simulink model "UDPKommunikation"  (Simulink 8.6)
settings: Solver=FixedStepAuto  StartTime=0.0  StopTime=inf  FixedStep=0.1  RelTol=1e-3
libraries: xpcutilitieslib x10, xpcrtudplib x10
settings Model: Creator=atlabor  LastModifiedBy=atlabor
settings DataIOCC: SaveFormat=Dataset  SignalLoggingSaveFormat=Dataset
settings OptimizationCC: ExpressionDepthLimit=128
settings DebuggingCC: UnderspecifiedInitializationDetection=Simplified  MergeDetectMultiDrivingBlocksExec=error  SolverPrmCheckMsg=none  FcnCallInpInsideContextMsg=EnableAllAsError  StateNameClashWarn=none
settings HardwareCC: ProdBitPerPointer=64  ProdLargestAtomicFloat=Float  ProdIntDivRoundTo=Zero  ProdEndianess=LittleEndian  ProdWordSize=64  ProdHWDeviceType=Intel->x86-64 (Windows64)
settings GRTTargetCC: GeneratePreprocessorConditionals=Use local settings  CombineOutputUpdateFcns=on  GRTInterface=off

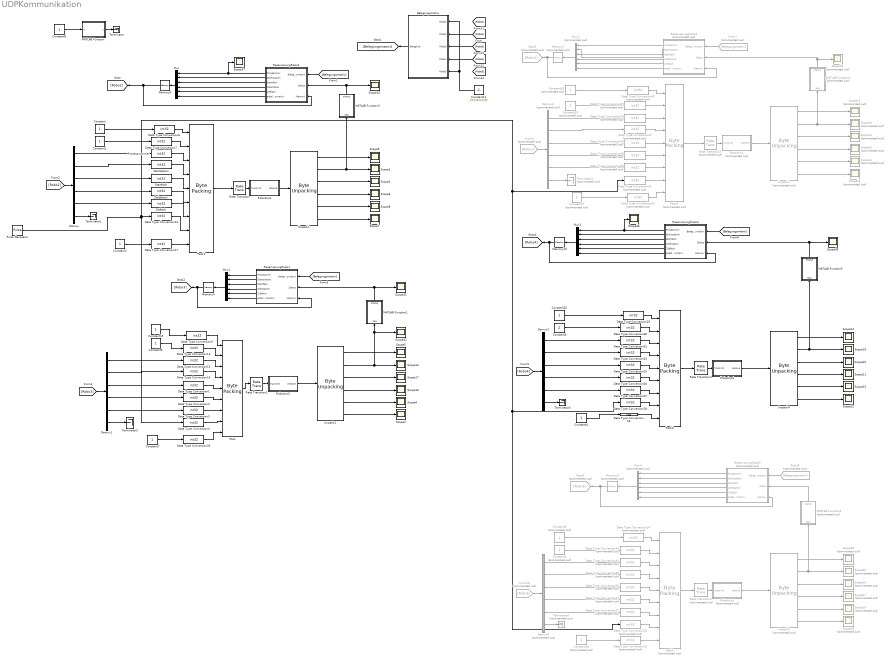
== system UDPKommunikation ==
  Belegungsmatrix : MATLAB Function  TreatAsAtomicUnit=on
  Constant{,1..2,4,7..9,15,25} (9 alike) : Constant
  Constant{5..6,10,17,28..29} (6 alike) : Constant  Commented=on
  Constant11 : Constant  Value=[0;0;0;0;0;0]
  Constant3 : Constant  Value=2
  Data Type Conversion{1..7,13..18,25..33} (22 alike) : DataTypeConversion  OutDataTypeStr=int32
  Data Type Conversion{19..24,34..45} (18 alike) : DataTypeConversion  Commented=on  OutDataTypeStr=int32
  Demux : Demux  Outputs=6
  Demux1 : Demux  Outputs=6
  Demux2 : Demux  Outputs=6
  Demux3 : Demux  Commented=on  Outputs=6
  Demux4 : Demux  Commented=on  Outputs=6
  From10 : From  Commented=on  GotoTag=Robo5
  From6 : From  Commented=on  GotoTag=Robo1
  From7 : From  Commented=on  GotoTag=Belegungsmatrix
  From9 : From  Commented=on  GotoTag=Belegungsmatrix
  Goto3 : Goto  Commented=on  GotoTag=Robo1
  Goto5 : Goto  Commented=on  GotoTag=Robo5
  MATLAB Function : MATLAB Function  TreatAsAtomicUnit=on
  MATLAB Function1 : MATLAB Function  TreatAsAtomicUnit=on
  MATLAB Function2 : MATLAB Function  Commented=on  TreatAsAtomicUnit=on
  MATLAB Function3 : MATLAB Function  TreatAsAtomicUnit=on
  MATLAB Function4 : MATLAB Function  Commented=on  TreatAsAtomicUnit=on
  MATLAB Function5 : MATLAB Function  TreatAsAtomicUnit=on
  Memory10 : Memory
  Memory4 : Memory
  Memory5 : Memory
  Memory7 : Memory  Commented=on
  Memory9 : Memory  Commented=on
  Mux : Mux  Inputs=6
  Mux1 : Mux  Inputs=6
  Mux2 : Mux  Commented=on  Inputs=6
  Mux3 : Mux  Inputs=6
  Mux4 : Mux  Commented=on  Inputs=6
  Pack : xpcutilitieslib/Byte Packing   MaskPackedDataType=uint8  MaskUnpackedDataTypes={'int32','int32','int32','int32','int32','int32','int32','int32','int32'}  MaskAlignment=1
  Pack1 : xpcutilitieslib/Byte Packing   Commented=on  MaskPackedDataType=uint8  MaskUnpackedDataTypes={'int32','int32','int32','int32','int32','int32','int32','int32','int32'}  MaskAlignment=1
  Pack2 : xpcutilitieslib/Byte Packing   MaskPackedDataType=uint8  MaskUnpackedDataTypes={'int32','int32','int32','int32','int32','int32','int32','int32','int32'}  MaskAlignment=1
  Pack3 : xpcutilitieslib/Byte Packing   MaskPackedDataType=uint8  MaskUnpackedDataTypes={'int32','int32','int32','int32','int32','int32','int32','int32','int32'}  MaskAlignment=1
  Pack4 : xpcutilitieslib/Byte Packing   Commented=on  MaskPackedDataType=uint8  MaskUnpackedDataTypes={'int32','int32','int32','int32','int32','int32','int32','int32','int32'}  MaskAlignment=1
  Prozessnummer : DataTypeConversion  OutDataTypeStr=int32
  Pulse Generator : DiscretePulseGenerator  PulseType=Time based  Amplitude=3  Period=1  PulseWidth=50
  Rate Transition : RateTransition  OutPortSampleTime=0.5
  Rate Transition1 : RateTransition  OutPortSampleTime=0.1
  Rate Transition2 : RateTransition  Commented=on  OutPortSampleTime=0.5
  Rate Transition3 : RateTransition  OutPortSampleTime=0.5
  Rate Transition4 : RateTransition  Commented=on  OutPortSampleTime=0.5
  ReservierungRobo1 : MATLAB Function  TreatAsAtomicUnit=on
  ReservierungRobo2 : MATLAB Function  TreatAsAtomicUnit=on
  ReservierungRobo3 : MATLAB Function  Commented=on  TreatAsAtomicUnit=on
  ReservierungRobo4 : MATLAB Function  TreatAsAtomicUnit=on
  ReservierungRobo5 : MATLAB Function  Commented=on  TreatAsAtomicUnit=on
  Robotino1 : Subsystem  Commented=on  TreatAsAtomicUnit=on
  Robotino2 : Subsystem  TreatAsAtomicUnit=on
  Robotino3 : Subsystem  TreatAsAtomicUnit=on
  Robotino4 : Subsystem  TreatAsAtomicUnit=on
  Robotino5 : Subsystem  Commented=on  TreatAsAtomicUnit=on
  Scope{1..9,16..24,31..33,35..37} (24 alike) : Scope
  Scope{10..15,25..30,34} (13 alike) : Scope  Commented=on
  Startfach : DataTypeConversion  OutDataTypeStr=int32
  Startstation : DataTypeConversion  OutDataTypeStr=int32
  Terminator{,1..3} (4 alike) : Terminator
  Terminator4 : Terminator  Commented=on
  Terminator5 : Terminator  Commented=on
  Unpack1 : xpcutilitieslib/Byte Unpacking   MaskUnpackedDataTypes={'uint32','uint32','uint32','uint32','uint32','uint32'}  MaskUnpackedDataSizes={1, 1,1,1,1,1}  MaskAlignment=1
  Unpack2 : xpcutilitieslib/Byte Unpacking   MaskUnpackedDataTypes={'uint32','uint32','uint32','uint32','uint32','uint32'}  MaskUnpackedDataSizes={1, 1,1,1,1,1}  MaskAlignment=1
  Unpack3 : xpcutilitieslib/Byte Unpacking   Commented=on  MaskUnpackedDataTypes={'uint32','uint32','uint32','uint32','uint32','uint32'}  MaskUnpackedDataSizes={1, 1,1,1,1,1}  MaskAlignment=1
  Unpack4 : xpcutilitieslib/Byte Unpacking   MaskUnpackedDataTypes={'uint32','uint32','uint32','uint32','uint32','uint32'}  MaskUnpackedDataSizes={1, 1,1,1,1,1}  MaskAlignment=1
  Unpack5 : xpcutilitieslib/Byte Unpacking   Commented=on  MaskUnpackedDataTypes={'uint32','uint32','uint32','uint32','uint32','uint32'}  MaskUnpackedDataSizes={1, 1,1,1,1,1}  MaskAlignment=1
  Zielfach : DataTypeConversion  OutDataTypeStr=int32
  Zielstation : DataTypeConversion  OutDataTypeStr=int32
  wires:
  Constant/1 -> Data Type Conversion6/1
  Pack2/1 -> Rate Transition/1
  Data Type Conversion6/1 -> Pack2/1
  Robotino2/1(receive) -> Unpack1/1
  Data Type Conversion7/1 -> Pack2/2
  Prozessnummer/1 -> Pack2/3
  Startstation/1 -> Pack2/4
  Startfach/1 -> Pack2/5
  Zielstation/1 -> Pack2/6
  Data Type Conversion13/1 -> Pack2/8
  Zielfach/1 -> Pack2/7
  Constant1/1 -> Data Type Conversion7/1
  Rate Transition/1 -> Robotino2/1(transmit)
  Constant8/1 -> MATLAB Function/1(u)
  MATLAB Function/1(y) -> Terminator/1
  Robotino3/1(receive) -> Unpack2/1
  Rate Transition1/1 -> Robotino3/1(transmit)
  Rate Transition2/1 -> Robotino1/1(transmit)
  Pack/1 -> Rate Transition1/1
  Data Type Conversion5/1 -> Pack/1
  Data Type Conversion14/1 -> Pack/2
  Data Type Conversion15/1 -> Pack/3
  Data Type Conversion16/1 -> Pack/4
  Data Type Conversion1/1 -> Pack/5
  Data Type Conversion2/1 -> Pack/6
  Data Type Conversion4/1 -> Pack/8
  Data Type Conversion3/1 -> Pack/7
  Constant9/1 -> Data Type Conversion14/1
  Pack4/1 -> Rate Transition2/1
  Constant15/1 -> Data Type Conversion5/1
  Rate Transition3/1 -> Robotino4/1(transmit)
  Pack3/1 -> Rate Transition3/1
  Data Type Conversion29/1 -> Pack3/1
  Data Type Conversion30/1 -> Pack3/2
  Data Type Conversion31/1 -> Pack3/3
  Data Type Conversion32/1 -> Pack3/4
  Data Type Conversion25/1 -> Pack3/5
  Data Type Conversion26/1 -> Pack3/6
  Data Type Conversion28/1 -> Pack3/8
  Data Type Conversion27/1 -> Pack3/7
  Constant25/1 -> Data Type Conversion29/1
  Constant3/1 -> Data Type Conversion30/1
  Unpack2/1 -> Scope5/1
  Unpack2/3 -> Scope17/1
  Unpack2/4 -> Scope18/1
  Unpack2/5 -> Scope4/1
  Unpack2/6 -> Scope2/1
  Data Type Conversion33/1 -> Pack/9
  Constant7/1 -> Data Type Conversion33/1
  Data Type Conversion42/1 -> Pack4/1
  Data Type Conversion35/1 -> Pack4/2
  Data Type Conversion36/1 -> Pack4/3
  Data Type Conversion37/1 -> Pack4/4
  Data Type Conversion34/1 -> Pack4/5
  Data Type Conversion38/1 -> Pack4/6
  Data Type Conversion41/1 -> Pack4/8
  Data Type Conversion39/1 -> Pack4/7
  Constant29/1 -> Data Type Conversion35/1
  Data Type Conversion40/1 -> Pack4/9
  Constant17/1 -> Data Type Conversion40/1
  Unpack1/1 -> Scope9/1
  Unpack1/2 -> MATLAB Function3/1(new), Scope1/1
  Unpack1/3 -> Scope3/1
  Unpack1/4 -> Scope6/1
  Unpack1/5 -> Scope8/1
  Unpack1/6 -> Scope7/1
  Robotino1/1(receive) -> Unpack3/1
  Unpack3/1 -> Scope15/1
  Unpack3/2 -> MATLAB Function2/1(new), Scope10/1
  Unpack3/3 -> Scope11/1
  Unpack3/4 -> Scope12/1
  Unpack3/5 -> Scope14/1
  Unpack3/6 -> Scope13/1
  Robotino4/1(receive) -> Unpack4/1
  Unpack4/1 -> Scope24/1
  Unpack4/3 -> Scope20/1
  Unpack4/4 -> Scope21/1
  Unpack4/5 -> Scope23/1
  Unpack4/6 -> Scope22/1
  Constant28/1 -> Data Type Conversion42/1
  Unpack4/2 -> MATLAB Function5/1(new), Scope19/1
  Data Type Conversion17/1 -> Pack2/9
  Constant2/1 -> Data Type Conversion17/1
  Data Type Conversion18/1 -> Pack3/9
  Constant4/1 -> Data Type Conversion18/1
  MATLAB Function3/1(status) -> ReservierungRobo2/2(Status), Scope33/1
  Rate Transition4/1 -> Robotino5/1(transmit)
  Pack1/1 -> Rate Transition4/1
  Data Type Conversion24/1 -> Pack1/1
  Data Type Conversion43/1 -> Pack1/2
  Data Type Conversion44/1 -> Pack1/3
  Data Type Conversion45/1 -> Pack1/4
  Data Type Conversion20/1 -> Pack1/5
  Data Type Conversion21/1 -> Pack1/6
  Data Type Conversion23/1 -> Pack1/8
  Data Type Conversion22/1 -> Pack1/7
  Constant5/1 -> Data Type Conversion24/1
  Constant6/1 -> Data Type Conversion43/1
  Pulse Generator/1 -> Data Type Conversion13/1, Data Type Conversion28/1, Data Type Conversion23/1, Data Type Conversion41/1, Data Type Conversion4/1
  Robotino5/1(receive) -> Unpack5/1
  Unpack5/1 -> Scope30/1
  Unpack5/3 -> Scope26/1
  Unpack5/4 -> Scope27/1
  Unpack5/5 -> Scope29/1
  Unpack5/6 -> Scope28/1
  Data Type Conversion19/1 -> Pack1/9
  Constant10/1 -> Data Type Conversion19/1
  ReservierungRobo2/1(Prozessnmr) -> Scope37/1, Mux/1
  ReservierungRobo2/2(Startstation) -> Mux/2
  ReservierungRobo2/3(Startfach) -> Mux/3
  ReservierungRobo2/4(Zielstation) -> Mux/4
  ReservierungRobo2/5(Zielfach) -> Mux/5
  ReservierungRobo2/6(enableBelegungsmatrix) -> Mux/6
  Belegungsmatrix/1(BelegOut) -> [Belegungsmatrix]
  [Belegungsmatrix] -> ReservierungRobo2/1(Belegungsmatrix)
  [Robo2] -> Demux/1
  Demux/1 -> Prozessnummer/1
  Demux/2 -> Startstation/1
  Demux/3 -> Startfach/1
  Demux/4 -> Zielstation/1
  Demux/5 -> Zielfach/1
  Demux/6 -> Terminator1/1
  Unpack2/2 -> MATLAB Function1/1(new), Scope32/1, Scope16/1
  ReservierungRobo1/1(Prozessnmr) -> Mux1/1
  ReservierungRobo1/2(Startstation) -> Mux1/2
  ReservierungRobo1/3(Startfach) -> Mux1/3
  ReservierungRobo1/4(Zielstation) -> Mux1/4
  ReservierungRobo1/5(Zielfach) -> Mux1/5
  ReservierungRobo1/6(enableBelegungsmatrix) -> Mux1/6
  [Belegungsmatrix] -> ReservierungRobo1/1(Belegungsmatrix)
  [Robo3] -> Demux1/1
  Demux1/1 -> Data Type Conversion15/1
  Demux1/2 -> Data Type Conversion16/1
  Demux1/3 -> Data Type Conversion1/1
  Demux1/4 -> Data Type Conversion2/1
  Demux1/5 -> Data Type Conversion3/1
  Demux1/6 -> Terminator2/1
  [Robo4] -> Demux2/1
  Demux2/1 -> Data Type Conversion31/1
  Demux2/2 -> Data Type Conversion32/1
  Demux2/3 -> Data Type Conversion25/1
  Demux2/4 -> Data Type Conversion26/1
  Demux2/5 -> Data Type Conversion27/1
  Demux2/6 -> Terminator3/1
  From6/1 -> Demux3/1
  Demux3/1 -> Data Type Conversion36/1
  Demux3/2 -> Data Type Conversion37/1
  Demux3/3 -> Data Type Conversion34/1
  Demux3/4 -> Data Type Conversion38/1
  Demux3/5 -> Data Type Conversion39/1
  Demux3/6 -> Terminator4/1
  MATLAB Function2/1(status) -> ReservierungRobo3/2(Status), Scope34/1
  ReservierungRobo3/1(Prozessnmr) -> Mux2/1
  ReservierungRobo3/2(Startstation) -> Mux2/2
  ReservierungRobo3/3(Startfach) -> Mux2/3
  ReservierungRobo3/4(Zielstation) -> Mux2/4
  ReservierungRobo3/5(Zielfach) -> Mux2/5
  ReservierungRobo3/6(enableBelegungsmatrix) -> Mux2/6
  From7/1 -> ReservierungRobo3/1(Belegungsmatrix)
  MATLAB Function5/1(status) -> ReservierungRobo4/2(Status), Scope35/1
  ReservierungRobo4/1(Prozessnmr) -> Scope36/1, Mux3/1
  ReservierungRobo4/2(Startstation) -> Mux3/2
  ReservierungRobo4/3(Startfach) -> Mux3/3
  ReservierungRobo4/4(Zielstation) -> Mux3/4
  ReservierungRobo4/5(Zielfach) -> Mux3/5
  ReservierungRobo4/6(enableBelegungsmatrix) -> Mux3/6
  [Belegungsmatrix] -> ReservierungRobo4/1(Belegungsmatrix)
  Unpack5/2 -> MATLAB Function4/1(new), Scope25/1
  MATLAB Function4/1(status) -> ReservierungRobo5/2(Status)
  ReservierungRobo5/1(Prozessnmr) -> Mux4/1
  ReservierungRobo5/2(Startstation) -> Mux4/2
  ReservierungRobo5/3(Startfach) -> Mux4/3
  ReservierungRobo5/4(Zielstation) -> Mux4/4
  ReservierungRobo5/5(Zielfach) -> Mux4/5
  ReservierungRobo5/6(enableBelegungsmatrix) -> Mux4/6
  From9/1 -> ReservierungRobo5/1(Belegungsmatrix)
  From10/1 -> Demux4/1
  Demux4/1 -> Data Type Conversion44/1
  Demux4/2 -> Data Type Conversion45/1
  Demux4/3 -> Data Type Conversion20/1
  Demux4/4 -> Data Type Conversion21/1
  Demux4/5 -> Data Type Conversion22/1
  Demux4/6 -> Terminator5/1
  Mux/1 -> Memory5/1
  Memory5/1 -> ReservierungRobo2/3(Memory), [Robo2]
  Memory7/1 -> ReservierungRobo3/3(Memory), Goto3/1
  Mux2/1 -> Memory7/1
  Mux3/1 -> Memory10/1
  Memory10/1 -> ReservierungRobo4/3(Memory), [Robo4]
  Mux1/1 -> Memory4/1
  Memory4/1 -> ReservierungRobo1/3(Memory), [Robo3]
  MATLAB Function1/1(status) -> ReservierungRobo1/2(Status), Scope31/1
  [Robo3] -> Belegungsmatrix/3(Robo3)
  Memory9/1 -> ReservierungRobo5/3(Memory), Goto5/1
  Mux4/1 -> Memory9/1
  [Robo4] -> Belegungsmatrix/4(Robo4)
  Constant11/1 -> Belegungsmatrix/5(Robo5), Belegungsmatrix/1(Robo1)
  [Robo2] -> Belegungsmatrix/2(Robo2)

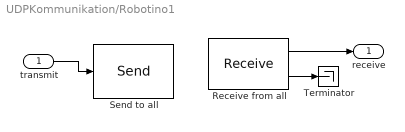
== system UDPKommunikation/Robotino1 ==
  transmit : Inport
  Receive from all : xpcrtudplib/Legacy UDP/Receive   ipAddress=192.168.0.11  ipPort=25010  width=24  vblLen=off  sampletime=-1
  Send to all : xpcrtudplib/Legacy UDP/Send   ipAddress=192.168.0.11  ipPort=25011  localPort=-1  vblLen=off  sampletime=-1
  Terminator : Terminator
  receive : Outport
  wires:
  transmit/1 -> Send to all/1
  Receive from all/2 -> Terminator/1
  Receive from all/1 -> receive/1

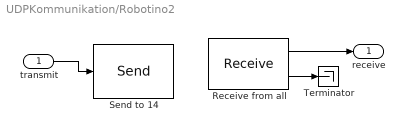
== system UDPKommunikation/Robotino2 ==
  transmit : Inport
  Receive from all : xpcrtudplib/Legacy UDP/Receive   ipAddress=192.168.0.12  ipPort=25020  width=24  vblLen=off  sampletime=-1
  Send to 14 : xpcrtudplib/Legacy UDP/Send   ipAddress=192.168.0.12  ipPort=25012  localPort=-1  vblLen=off  sampletime=-1
  Terminator : Terminator
  receive : Outport
  wires:
  transmit/1 -> Send to 14/1
  Receive from all/2 -> Terminator/1
  Receive from all/1 -> receive/1

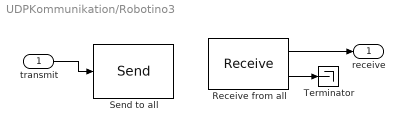
== system UDPKommunikation/Robotino3 ==
  transmit : Inport
  Receive from all : xpcrtudplib/Legacy UDP/Receive   ipAddress=192.168.0.13  ipPort=25030  width=24  vblLen=off  sampletime=-1
  Send to all : xpcrtudplib/Legacy UDP/Send   ipAddress=192.168.0.13  ipPort=25013  localPort=9  vblLen=off  sampletime=-1
  Terminator : Terminator
  receive : Outport
  wires:
  Receive from all/1 -> receive/1
  Receive from all/2 -> Terminator/1
  transmit/1 -> Send to all/1

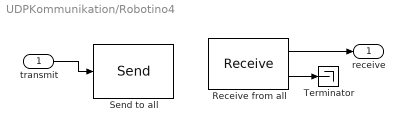
== system UDPKommunikation/Robotino4 ==
  transmit : Inport
  Receive from all : xpcrtudplib/Legacy UDP/Receive   ipAddress=192.168.0.14  ipPort=25040  width=24  vblLen=off  sampletime=-1
  Send to all : xpcrtudplib/Legacy UDP/Send   ipAddress=192.168.0.14  ipPort=25014  localPort=-1  vblLen=off  sampletime=-1
  Terminator : Terminator
  receive : Outport
  wires:
  transmit/1 -> Send to all/1
  Receive from all/2 -> Terminator/1
  Receive from all/1 -> receive/1

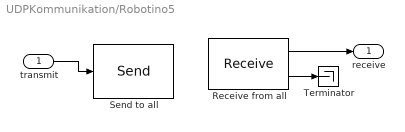
== system UDPKommunikation/Robotino5 ==
  transmit : Inport
  Receive from all : xpcrtudplib/Legacy UDP/Receive   ipAddress=192.168.0.211  ipPort=25050  width=24  vblLen=off  sampletime=-1
  Send to all : xpcrtudplib/Legacy UDP/Send   ipAddress=192.168.0.211  ipPort=25015  localPort=-1  vblLen=off  sampletime=-1
  Terminator : Terminator
  receive : Outport
  wires:
  transmit/1 -> Send to all/1
  Receive from all/2 -> Terminator/1
  Receive from all/1 -> receive/1

== matlab function MATLAB Function1 ==
  data: new input double; status output double
function status = fcn(new)
persistent old 
persistent firstRun
status =1;
if isempty(firstRun)
    firstRun = 1;
    old = 1;
end

if (old ~= new && new == 0)
    status = 0;
else 
    status = 1;
end
old = double(new);

== matlab function MATLAB Function ==
  data: u input double; y output double
function y = fcn(u)
%#codegen
pause(0.1)
y = u;

== matlab function ReservierungRobo1 ==
  data: Belegungsmatrix input double; Status input double; Prozessnmr output double; Startstation output double; Startfach output double; Zielstation output double; Zielfach output double; enableBelegungsmatrix output double; Memory input double
function  [Prozessnmr,Startstation,Startfach,Zielstation,Zielfach,enableBelegungsmatrix]= fcn(Belegungsmatrix,Status,Memory)
%#codegen
persistent tryAgain 
persistent ProzessnrCount
if isempty(ProzessnrCount)
    ProzessnrCount =1;
end
if Status==0 
    tryAgain = 1;
    Startfach       = 1;
    Startstation    = 1;
    Zielstation     = 7;
    Zielfach        = 1;
    while tryAgain
        %Startfach
        RoboStartStationBumbar      = randi(8,1)-1;
        RoboStartfachBumbar         = randi(2,1)-1;
        if Belegungsmatrix(RoboStartfachBumbar+1,RoboStartStationBumbar+1)== 1
                Startstation    = RoboStartStationBumbar;
                Startfach       = RoboStartfachBumbar;
                tryAgain = 0;
        end
    end
    tryAgain = 1;
    while tryAgain
        %Zielfach
        RoboZielStationBumbar      = randi(8,1)-1;
        RoboZielfachBumbar         = randi(2,1)-1;
        if Belegungsmatrix(RoboZielfachBumbar+1,RoboZielStationBumbar+1)== 0
                Zielstation    = RoboZielStationBumbar;
                Zielfach       = RoboZielfachBumbar;
                tryAgain = 0;
        end
    end
    if ProzessnrCount == 1
        Startfach       = 1;
        Startstation    = 0;
        Zielstation     = 7;
        Zielfach        = 1;
    end
    enableBelegungsmatrix = 1;
    Prozessnmr = ProzessnrCount +1;
    ProzessnrCount = Prozessnmr;
    
else
    Prozessnmr      = Memory(1);
    Startstation    = Memory(2);
    Startfach       = Memory(3);
    Zielstation     = Memory(4);
    Zielfach        = Memory(5);
    enableBelegungsmatrix = 0;
end
end

== matlab function MATLAB Function3 ==
  data: new input double; status output double
function status = fcn(new)
persistent old 
persistent firstRun
status =1;
if isempty(firstRun)
    firstRun = 1;
    old = 1;
end

if (old ~= new && new == 0)
    status = 0;
else 
    status = 1;
end
old = double(new);

== matlab function MATLAB Function4 ==
  data: new input double; status output double
function status = fcn(new)
persistent old 
persistent firstRun
status =1;
if isempty(firstRun)
    firstRun = 1;
    old = 1;
end

if (old ~= new && new == 0)
    status = 0;
else 
    status = 1;
end
old = double(new);

== matlab function ReservierungRobo2 ==
  data: Belegungsmatrix input double; Status input double; Prozessnmr output double; Startstation output double; Startfach output double; Zielstation output double; Zielfach output double; enableBelegungsmatrix output double; Memory input double
function  [Prozessnmr,Startstation,Startfach,Zielstation,Zielfach,enableBelegungsmatrix]= fcn(Belegungsmatrix,Status,Memory)
%#codegen
persistent tryAgain 
persistent ProzessnrCount
if isempty(ProzessnrCount)
    ProzessnrCount =1;
end
if Status==0 
        
    tryAgain = 1;
    Startfach       = 1;
    Startstation    = 1;
    Zielstation     = 7;
    Zielfach        = 1;
    while tryAgain
        %Startfach
        RoboStartStationBumbar      = randi(8,1)-1;
        RoboStartfachBumbar         = randi(2,1)-1;
        if Belegungsmatrix(RoboStartfachBumbar+1,RoboStartStationBumbar+1)== 1
                Startstation    = RoboStartStationBumbar;
                Startfach       = RoboStartfachBumbar;
                tryAgain = 0;
        end
    end
    tryAgain = 1;
    while tryAgain
        %Zielfach
        RoboZielStationBumbar      = randi(8,1)-1;
        RoboZielfachBumbar         = randi(2,1)-1;
        if Belegungsmatrix(RoboZielfachBumbar+1,RoboZielStationBumbar+1)== 0
                Zielstation    = RoboZielStationBumbar;
                Zielfach       = RoboZielfachBumbar;
                tryAgain = 0;
        end
    end
    if ProzessnrCount == 1
    Startfach       = 0;
    Startstation    = 0;
    Zielstation     = 7;
    Zielfach        = 0;
    end
    enableBelegungsmatrix = 1;
    Prozessnmr = ProzessnrCount +1;
    ProzessnrCount = Prozessnmr;
    
else
    Prozessnmr      = Memory(1);
    Startstation    = Memory(2);
    Startfach       = Memory(3);
    Zielstation     = Memory(4);
    Zielfach        = Memory(5);
    enableBelegungsmatrix = 0;
end
end

== matlab function Belegungsmatrix ==
  data: Robo1 input double; Robo2 input double; Robo3 input double; Robo4 input double; Robo5 input double; BelegOut output double size=[2 8]
function BelegOut = fcn(Robo1,Robo2,Robo3,Robo4,Robo5)

persistent Belegungsmatrix
persistent fuckyou

persistent Robo1StartStationOld
persistent Robo1StartfachOld
persistent Robo1ZielStationOld
persistent Robo1ZielfachOld

persistent Robo2StartStationOld
persistent Robo2StartfachOld
persistent Robo2ZielStationOld
persistent Robo2ZielfachOld

persistent Robo3StartStationOld
persistent Robo3StartfachOld
persistent Robo3ZielStationOld
persistent Robo3ZielfachOld

persistent Robo4StartStationOld
persistent Robo4StartfachOld
persistent Robo4ZielStationOld
persistent Robo4ZielfachOld

persistent Robo5StartStationOld
persistent Robo5StartfachOld
persistent Robo5ZielStationOld
persistent Robo5ZielfachOld

if isempty(fuckyou)
    fuckyou =1;
    Belegungsmatrix = [ones(2,2), zeros(2,6)];
    Robo1StartStationOld = 1;
    Robo1StartfachOld    = 1;
    Robo1ZielStationOld  = 7;
    Robo1ZielfachOld     = 0;
    
    Robo2StartStationOld = 1;
    Robo2StartfachOld    = 1;
    Robo2ZielStationOld  = 7;
    Robo2ZielfachOld     = 1;
    
    Robo3StartStationOld = 1;
    Robo3StartfachOld    = 1;
    Robo3ZielStationOld  = 6;
    Robo3ZielfachOld     = 0;
    
    Robo4StartStationOld = 1;
    Robo4StartfachOld    = 1;
    Robo4ZielStationOld  = 6;
    Robo4ZielfachOld     = 1;
    
    Robo5StartStationOld = 1;
    Robo5StartfachOld    = 1;
    Robo5ZielStationOld  = 7;
    Robo5ZielfachOld     = 1;
end
%Roboter 1
Robo1StartStation   = Robo1(2);
Robo1Startfach      = Robo1(3);
Robo1ZielStation    = Robo1(4);
Robo1Zielfach       = Robo1(5);
Robo1Enable         = Robo1(6);

%Roboter 2
Robo2StartStation   = Robo2(2);
Robo2Startfach      = Robo2(3);
Robo2ZielStation    = Robo2(4);
Robo2Zielfach       = Robo2(5);
Robo2Enable         = Robo2(6);
%Roboter 3
Robo3StartStation   = Robo3(2);
Robo3Startfach      = Robo3(3);
Robo3ZielStation    = Robo3(4);
Robo3Zielfach       = Robo3(5);
Robo3Enable         = Robo3(6);
%Roboter 4
Robo4StartStation   = Robo4(2);
Robo4Startfach      = Robo4(3);
Robo4ZielStation    = Robo4(4);
Robo4Zielfach       = Robo4(5);
Robo4Enable         = Robo4(6);

%Roboter 5
Robo5StartStation   = Robo5(2);
Robo5Startfach      = Robo5(3);
Robo5ZielStation    = Robo5(4);
Robo5Zielfach       = Robo5(5);
Robo5Enable         = Robo5(6);

if Robo1Enable == 1
    Belegungsmatrix(Robo1StartfachOld+1,Robo1StartStationOld+1) = 0;
    Belegungsmatrix(Robo1ZielfachOld+1,Robo1ZielStationOld+1)   = 1;
    Belegungsmatrix(Robo1Startfach+1,Robo1StartStation+1)       = 2;
    Belegungsmatrix(Robo1Zielfach+1,Robo1ZielStation+1)         = 2;

    Robo1StartfachOld   = Robo1Startfach;
    Robo1ZielfachOld    = Robo1Zielfach;
    Robo1StartStationOld= Robo1StartStation;
    Robo1ZielStationOld = Robo1ZielStation;

end
if Robo2Enable == 1
    Belegungsmatrix(Robo2StartfachOld+1,Robo2StartStationOld+1) = 0;
    Belegungsmatrix(Robo2ZielfachOld+1,Robo2ZielStationOld+1)   = 1;
    Belegungsmatrix(Robo2Startfach+1,Robo2StartStation+1)       = 2;
    Belegungsmatrix(Robo2Zielfach+1,Robo2ZielStation+1)         = 2;

    Robo2StartfachOld   = Robo2Startfach;
    Robo2ZielfachOld    = Robo2Zielfach;
    Robo2StartStationOld= Robo2StartStation;
    Robo2ZielStationOld = Robo2ZielStation;
end
if Robo3Enable == 1
    Belegungsmatrix(Robo3StartfachOld+1,Robo3StartStationOld+1) = 0;
    Belegungsmatrix(Robo3ZielfachOld+1,Robo3ZielStationOld+1)   = 1;
    Belegungsmatrix(Robo3Startfach+1,Robo3StartStation+1)       = 2;
    Belegungsmatrix(Robo3Zielfach+1,Robo3ZielStation+1)         = 2;

    Robo3StartfachOld   = Robo3Startfach;
    Robo3ZielfachOld    = Robo3Zielfach;
    Robo3StartStationOld= Robo3StartStation;
    Robo3ZielStationOld = Robo3ZielStation;
    
end
if Robo4Enable == 1
    Belegungsmatrix(Robo4StartfachOld+1,Robo4StartStationOld+1) = 0;
    Belegungsmatrix(Robo4ZielfachOld+1,Robo4ZielStationOld+1)   = 1;
    Belegungsmatrix(Robo4Startfach+1,Robo4StartStation+1)       = 2;
    Belegungsmatrix(Robo4Zielfach+1,Robo4ZielStation+1)         = 2;

    Robo4StartStationOld= Robo4StartStation;
    Robo4StartfachOld   = Robo4Startfach;
    Robo4ZielStationOld = Robo4ZielStation;
    Robo4ZielfachOld    = Robo4Zielfach;
    
end
if Robo5Enable == 1
    Belegungsmatrix(Robo5StartfachOld+1,Robo5StartStationOld+1) = 0;
    Belegungsmatrix(Robo5ZielfachOld+1,Robo5ZielStationOld+1)   = 1;
    Belegungsmatrix(Robo5Startfach+1,Robo5StartStation+1)       = 2;
    Belegungsmatrix(Robo5Zielfach+1,Robo5ZielStation+1)         = 2;

    Robo5StartfachOld   = Robo5Startfach;
    Robo5ZielfachOld    =  Robo5Zielfach;
    Robo5StartStationOld = Robo5StartStation;
    Robo5ZielStationOld = Robo5ZielStation;
end


if (Robo1Enable|Robo2Enable|Robo3Enable|Robo4Enable|Robo5Enable) == 1
    Ausgabe = [Belegungsmatrix(2,:);Belegungsmatrix(1,:)]
end
    Belegungsmatrix(1:2,1:2) = [ones(2,2)];
    Belegungsmatrix(1:2,7:8) = [zeros(2,2)];
BelegOut = Belegungsmatrix;

== matlab function MATLAB Function2 ==
  data: new input double; status output double
function status = fcn(new)
persistent old 
persistent firstRun
status =1;
if isempty(firstRun)
    firstRun = 1;
    old = 1;
end

if (old ~= new && new == 0)
    status = 0;
else 
    status = 1;
end
old = double(new);

== matlab function ReservierungRobo3 ==
  data: Belegungsmatrix input double; Status input double; Prozessnmr output double; Startstation output double; Startfach output double; Zielstation output double; Zielfach output double; enableBelegungsmatrix output double; Memory input double
function  [Prozessnmr,Startstation,Startfach,Zielstation,Zielfach,enableBelegungsmatrix]= fcn(Belegungsmatrix,Status,Memory)
%#codegen
persistent tryAgain 
persistent ProzessnrCount
if isempty(ProzessnrCount)
    ProzessnrCount =1;
end
if Status==0 
    tryAgain = 1;
    Startfach       = 1;
    Startstation    = 1;
    Zielstation     = 7;
    Zielfach        = 1;
    while tryAgain
        %Startfach
        RoboStartStationBumbar      = randi(8,1)-1;
        RoboStartfachBumbar         = randi(2,1)-1;
        if Belegungsmatrix(RoboStartfachBumbar+1,RoboStartStationBumbar+1)== 1
                Startstation    = RoboStartStationBumbar;
                Startfach       = RoboStartfachBumbar;
                tryAgain = 0;
        end
    end
    tryAgain = 1;
    while tryAgain
        %Zielfach
        RoboZielStationBumbar      = randi(8,1)-1;
        RoboZielfachBumbar         = randi(2,1)-1;
        if Belegungsmatrix(RoboZielfachBumbar+1,RoboZielStationBumbar+1)== 0
                Zielstation    = RoboZielStationBumbar;
                Zielfach       = RoboZielfachBumbar;
                tryAgain = 0;
        end
    end
    if ProzessnrCount == 1
        Startfach       = 0;
        Startstation    = 1;
        Zielstation     = 6;
        Zielfach        = 0;
    end
    enableBelegungsmatrix = 1;
    Prozessnmr = ProzessnrCount +1;
    ProzessnrCount = Prozessnmr;
    
else
    Prozessnmr      = Memory(1);
    Startstation    = Memory(2);
    Startfach       = Memory(3);
    Zielstation     = Memory(4);
    Zielfach        = Memory(5);
    enableBelegungsmatrix = 0;
end
end

== matlab function MATLAB Function5 ==
  data: new input double; status output double
function status = fcn(new)
persistent old 
persistent firstRun
status =1;
if isempty(firstRun)
    firstRun = 1;
    old = 1;
end

if (old ~= new && new == 0)
    status = 0;
else 
    status = 1;
end
old = double(new);

== matlab function ReservierungRobo4 ==
  data: Belegungsmatrix input double; Status input double; Prozessnmr output double; Startstation output double; Startfach output double; Zielstation output double; Zielfach output double; enableBelegungsmatrix output double; Memory input double
function  [Prozessnmr,Startstation,Startfach,Zielstation,Zielfach,enableBelegungsmatrix]= fcn(Belegungsmatrix,Status,Memory)
%#codegen
persistent tryAgain 
persistent ProzessnrCount
if isempty(ProzessnrCount)
    ProzessnrCount =1;
end
if Status==0 
    tryAgain = 1;
    Startfach       = 1;
    Startstation    = 1;
    Zielstation     = 7;
    Zielfach        = 1;
    while tryAgain
        %Startfach
        RoboStartStationBumbar      = randi(8,1)-1;
        RoboStartfachBumbar         = randi(2,1)-1;
        if Belegungsmatrix(RoboStartfachBumbar+1,RoboStartStationBumbar+1)== 1
                Startstation    = RoboStartStationBumbar;
                Startfach       = RoboStartfachBumbar;
                tryAgain = 0;
        end
    end
    tryAgain = 1;
    while tryAgain
        %Zielfach
        RoboZielStationBumbar      = randi(8,1)-1;
        RoboZielfachBumbar         = randi(2,1)-1;
        if Belegungsmatrix(RoboZielfachBumbar+1,RoboZielStationBumbar+1)== 0
                Zielstation    = RoboZielStationBumbar;
                Zielfach       = RoboZielfachBumbar;
                tryAgain = 0;
        end
    end
    if ProzessnrCount == 1
        Startfach       = 1;
        Startstation    = 1;
        Zielstation     = 6;
        Zielfach        = 1;
    end
    enableBelegungsmatrix = 1;
    Prozessnmr = ProzessnrCount +1;
    ProzessnrCount = Prozessnmr;
    
else
    Prozessnmr      = Memory(1);
    Startstation    = Memory(2);
    Startfach       = Memory(3);
    Zielstation     = Memory(4);
    Zielfach        = Memory(5);
    enableBelegungsmatrix = 0;
end
end

== matlab function ReservierungRobo5 ==
  data: Belegungsmatrix input double; Status input double; Prozessnmr output double; Startstation output double; Startfach output double; Zielstation output double; Zielfach output double; enableBelegungsmatrix output double; Memory input double
function  [Prozessnmr,Startstation,Startfach,Zielstation,Zielfach,enableBelegungsmatrix]= fcn(Belegungsmatrix,Status,Memory)
%#codegen
persistent tryAgain 
persistent ProzessnrCount
if isempty(ProzessnrCount)
    ProzessnrCount =1;
end
if Status==0 
    tryAgain = 1;
    Startfach       = 1;
    Startstation    = 1;
    Zielstation     = 7;
    Zielfach        = 1;
    while tryAgain
        %Startfach
        RoboStartStationBumbar      = randi(8,1)-1;
        RoboStartfachBumbar         = randi(2,1)-1;
        if Belegungsmatrix(RoboStartfachBumbar+1,RoboStartStationBumbar+1)== 1
                Startstation    = RoboStartStationBumbar;
                Startfach       = RoboStartfachBumbar;
                tryAgain = 0;
        end
    end
    tryAgain = 1;
    while tryAgain
        %Zielfach
        RoboZielStationBumbar      = randi(8,1)-1;
        RoboZielfachBumbar         = randi(2,1)-1;
        if Belegungsmatrix(RoboZielfachBumbar+1,RoboZielStationBumbar+1)== 0
                Zielstation    = RoboZielStationBumbar;
                Zielfach       = RoboZielfachBumbar;
                tryAgain = 0;
        end
    end

    enableBelegungsmatrix = 1;
    Prozessnmr = ProzessnrCount +1;
    ProzessnrCount = Prozessnmr;
    
else
    Prozessnmr      = Memory(1);
    Startstation    = Memory(2);
    Startfach       = Memory(3);
    Zielstation     = Memory(4);
    Zielfach        = Memory(5);
    enableBelegungsmatrix = 0;
end
end
